simulink model "Buck_boost"  (R2014a)
settings: Solver=ode23tb  SolverMode=SingleTasking  StartTime=0.0  StopTime=0.08  MaxStep=5e-6  RelTol=1e-3
libraries: powerlib x9, powerlib_meascontrol x1
settings Model: CovSFcnEnable=on  ExtModeTrigMode=oneshot  ExtModeArmWhenConnect=off  ExtModeAutoUpdateStatusClock=off  Creator=patrice  LastModifiedBy=DELL
settings DataIOCC: LimitDataPoints=off  SignalLoggingSaveFormat=ModelDataLogs  SignalLoggingName=sigsOut
settings OptimizationCC: BooleanDataType=off  InitFltsAndDblsToZero=on
settings DebuggingCC: SaveWithParameterizedLinksMsg=none  UnderspecifiedInitializationDetection=Classic  SignalResolutionControl=TryResolveAllWithWarning  SolverPrmCheckMsg=none  MultiTaskDSMMsg=warning  MultiTaskCondExecSysMsg=none  FcnCallInpInsideContextMsg=EnableAllAsWarning  FrameProcessingCompatibilityMsg=error
settings HardwareCC: TargetUnknown=on
settings RTWCC: TemplateMakefile=grt_unix.tmf
settings GRTTargetCC: TargetFcnLib=ansi_tfl_tmw.mat  CombineOutputUpdateFcns=off  GRTInterface=on
settings ConfigurationSet: Description=Simscape Multibody

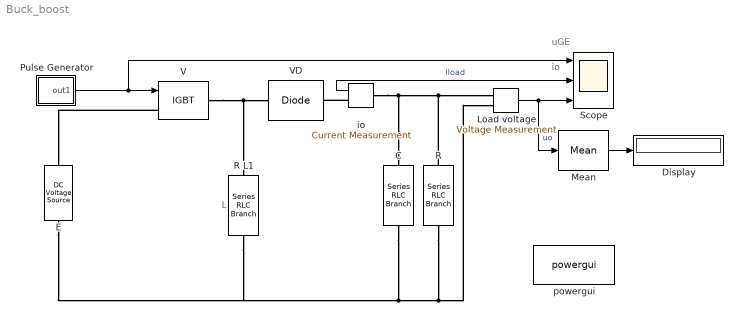
== system Buck_boost ==
  note: io
  note: uGE
  note: L
  C : powerlib/Elements/Series RLC Branch  LConnTagsString=__new0  RConnTagsString=__new0  BranchType=C  Resistance=0  Inductance=0  SetiL0=off  InitialCurrent=0  Capacitance=1e-3  Setx0=off  InitialVoltage=0  Measurements=None
  Display : Display
  E : powerlib/Electrical Sources/DC Voltage Source  Description=source block  Amplitude=100  Measurements=None
      settings: AttributesFormatString=%<Amplitude>V
  Load voltage : powerlib/Measurements/Voltage Measurement  Tag=PoWeRsYsTeMmEaSuReMeNt  PhasorSimulation=off  OutputType=Magnitude  PSBequivalent=0
  Mean : powerlib_meascontrol/Measurements/Mean  Freq=1000  Vinit=0  Ts=0  treatSBRowAsCol=off
  Pulse Generator : Subsystem  mask(Pulse Generator){period=1e-3, duty=50, amplitude=1, start=0}
      mask prompts: period "Period (secs):"; duty "Duty cycle (% of period):"; start "Start time:"
      mask help: Pulse Generator
      mask Help: Pulse generator which ensures pulse transitions are hit. Provides a vector of pulses when the height is entered as a vector.  Unmask to see how it works.
      mask Display: plot(0,0,100,100,[95,90,90,75,75,60,60,45,45,30,30,15,15,5],[25,25,75,75,25,25,75,75,25,25,75,75,25,25]);
  R : powerlib/Elements/Series RLC Branch  LConnTagsString=__new0  RConnTagsString=__new0  BranchType=R  Resistance=5  Inductance=0  SetiL0=off  InitialCurrent=0  Capacitance=inf  Setx0=off  InitialVoltage=0  Measurements=None
  R L1 : powerlib/Elements/Series RLC Branch  LConnTagsString=__new0  RConnTagsString=__new0  BranchType=L  Resistance=0  Inductance=5e-03  SetiL0=off  InitialCurrent=0  Capacitance=inf  Setx0=off  InitialVoltage=0  Measurements=None
  Scope : Scope  NumInputPorts=3
      settings: TimeRange=0.01  MaxDataPoints=500000  SaveToWorkspace=off  SaveName=ScopeData  YMin=-0.125~-7.65013~-138.15537  YMax=1.125~66.63916~15.36075  SampleTime=-1  DataFormat=Array
  V : powerlib/Power Electronics/IGBT  Ron=0.01  Lon=1e-6  Vf=1  Tf=1e-6  Tt=1e-6  IC=0  Rs=1000  Cs=1e-7  Measurements=off
      settings: AttributesFormatString=\n
  VD : powerlib/Power Electronics/Diode  Ron=0.01  Lon=1e-7  Vf=0.8  IC=0  UseSnubber=0  Rs=1000  Cs=0.1e-6  Measurements=off
  io : powerlib/Measurements/Current Measurement  Tag=PoWeRsYsTeMmEaSuReMeNt  PhasorSimulation=off  OutputType=Magnitude  PSBequivalent=0
  powergui : powerlib/powergui  Priority=1  SimulationMode=Continuous  SampleTime=50e-6  frequency=60  Iterations=50  frequencyindice=0  Pbase=100e6  ErrMax=1e-4  UnitsV=kV  UnitsW=MW  buscounter=0  FunctionMessages=off  echomessages=off  EnableUseOfTLC=off  CurrentSourceSwitches=off  DisableSnubberDevices=off  DisableRonSwitches=off  DisableVfSwitches=off  DisplayEquations=off  AutomaticDiscreteSolvers=off  SolverType=Tustin/Backward Euler (TBE)  Interpol=off  ExternalGateDelay=off  methode=off  Ts=100  x0status=blocks  SPID=on  SwTol=0  HookPort=off  NonlinearTolerance=1e-4  nMaxIteration=100  ContinueOnMaxIteration=off  RestoreLinks=warning  ResistiveCurrentMeasurement=off  Frange=[0:2:500]  Ylog=off  Xlog=on  ShowGrid=off  save=off  variable=ZData  structure=0  ZoomFFT=off  StartTime=0.0  cycles=1  DisplayStyle=1  fundamental=60  FreqAxis=off  MaxFrequency=1000  frequencyindicesteady=1  RmsSteady=1  display=off
  wires:
  io/1 -> Scope/2  "Iload"
  Pulse Generator/1(out1) -> Scope/1, V/1
  Mean/1 -> Display/1
  Load voltage/1 -> Mean/1, Scope/3  "uo"
  connections:
  io/LConn1 -- R/LConn1 -- Load voltage/LConn1 -- C/LConn1
  E/LConn1 -- R L1/RConn1 -- Load voltage/LConn2 -- R/RConn1 -- C/RConn1
  V/LConn1 -- E/RConn1
  V/RConn1 -- VD/RConn1 -- R L1/LConn1
  io/RConn1 -- VD/LConn1

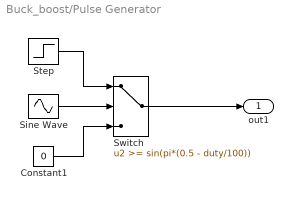
== system Buck_boost/Pulse Generator ==
  Constant1 : Constant  Value=0
  Sine Wave : Sin  Frequency=2*pi./period  Phase=-2*pi*(start./period + duty/200 - 1/4)  SampleTime=0
  Step : Step  Time=start  After=amplitude  SampleTime=0
  Switch : Switch  Threshold=sin(pi*(0.5 - duty/100))  SaturateOnIntegerOverflow=on  InputSameDT=on
  out1 : Outport  InitialOutput=0
  wires:
  Step/1 -> Switch/1
  Constant1/1 -> Switch/3
  Switch/1 -> out1/1
  Sine Wave/1 -> Switch/2
